simulink model "timercircuit"  (R2025b)
settings: Solver=VariableStepAuto  StartTime=0.0  StopTime=10.0  RelTol=1e-3
libraries: hdlsllib x1
settings Model: Creator=cyber  LastModifiedBy=cyber

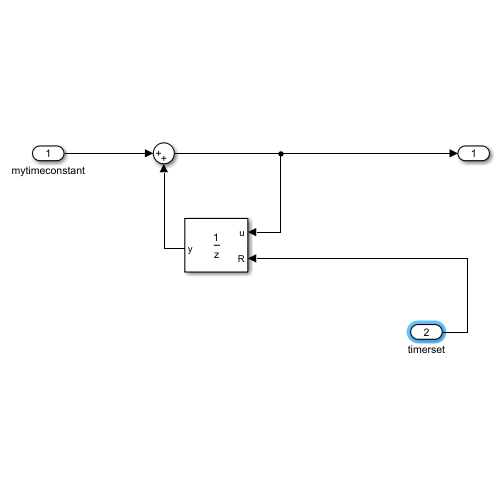
[thumbnail: Simulink's stored preview of the top-level diagram]
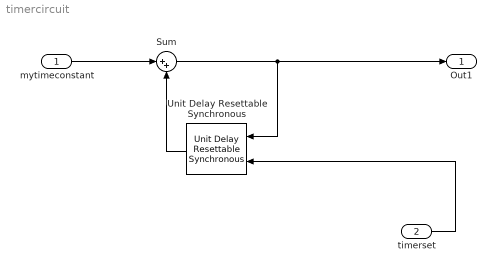
== system timercircuit ==
  mytimeconstant : Inport
  timerset : Inport  Port=2
  Sum : Sum  Inputs=|++
  Unit Delay Resettable Synchronous : hdlsllib/Discrete/Unit Delay Resettable Synchronous  InitialCondition=0.0  SampleTime=-1
  Out1 : Outport
  wires:
  Unit Delay Resettable Synchronous/1 -> Sum/2
  mytimeconstant/1 -> Sum/1
  Sum/1 -> Unit Delay Resettable Synchronous/1, Out1/1
  timerset/1 -> Unit Delay Resettable Synchronous/2
